simulink model "bh_2dof_NP_LGR_COMPONENT_model"  (R2017a)
settings: Solver=ode45  StartTime=0.0  StopTime=60  FixedStep=0.001  RelTol=1e-7  EnableMultiTasking=on
values from neighbouring files (symbols this model uses):
  theta1_0 = 0    [bh_SIMPARAMS_for_2dof_NP_Control_sim.m]
  theta1_dot_0 = 0    [bh_SIMPARAMS_for_2dof_NP_Control_sim.m]
  theta4_0 = 0    [bh_SIMPARAMS_for_2dof_NP_Control_sim.m]
  theta4_dot_0 = 0    [bh_SIMPARAMS_for_2dof_NP_Control_sim.m]
undefined symbols (not defined in the file or in its folder): b1_damp, b4_damp, g, L1x, L1y, L1z, mass1, mass4, Rturn
settings Model: Creator=bhorton  LastModifiedBy=bhorton
settings SolverCC: ZeroCrossAlgorithm=Adaptive
settings OptimizationCC: LifeSpan=inf
settings DebuggingCC: SFUnexpectedBacktrackingDiag=warning  SFNoUnconditionalDefaultTransitionDiag=warning  SFExecutionAtInitializationDiag=none
settings GRTTargetCC: TargetLangStandard=C89/C90 (ANSI)
settings ConfigComp: CovMetricSettings=dw  CovHtmlReporting=on  CovSaveCumulativeToWorkspaceVar=on  CovSaveSingleToWorkspaceVar=on  CovExternalEMLEnable=off
settings SimscapeCC: SimscapeLogDataHistory=10000  SelectedTab=Simscape Multibody
settings ExplorerConfigSet: InternalSimMechanicsExplorerSettings="<ExplorerConfiguration><canonicalview>default</canonicalview><AnimationSetting><BasePlaybackSpeed>1.0</BasePlaybackSpeed><PlaybackSpeedFactor>1.0</PlaybackSpeedFactor></AnimationSetting><TilePanel><TileInfo><Tiles Columns=\"2\" Count=\"4\" Rows=\"2\"><Column Left=\"2\" Weight=\"0.4997\"/><Column Left=\"761\" Weight=\"0.5003\"/><Column Left=\"1521\"/><Row Top=\"2\" Weight=\"0.4995\"/><Row Top=\"476\" Weight=\"0.5005\"/><Row Top=\"951\"/><Tile Height=\"1\" Width=\"1\" X=\"0\" Y=\"0\"/><Tile Height=\"1\" Width=\"1\" X=\"0\" Y=\"1\"/><Tile Height=\"1\" Width=\"1\" X=\"1\" Y=\"0\"/><Tile Height=\"1\" Width=\"1\" X=\"1\" Y=\"1\"/></Tiles></TileInfo><SceneInfo><SceneViewer><BGColor><R>0.60000002384185791</R><G>0.60000002384185791</G><B>0.60000002384185791</B></BGColor><Camera><DoPerspective>off</DoPerspective><Position><X>0</X><Y>-1.4608099072997489</Y><Z>-0.57289350032806285</Z></Position><Center><X>0</X><Y>0.46399667501581587</Y><Z>-0.57289350032806285</Z></Center><Up><X>0</X><Y>-0</Y><Z>1</Z></Up><ViewLimDist>1</ViewLimDist><YLim>0.6047525054216385</YLim><XLim>0.97540726680909429</XLim></Camera></SceneViewer><SceneViewer><BGColor><R>0.60000002384185791</R><G>0.60000002384185791</G><B>0.60000002384185791</B></BGColor><Camera><DoPerspective>off</DoPerspective><Position><X>0.015927683572912424</X><Y>0.0885583895662721</Y><Z>1.3002562391579151</Z></Position><Center><X>0.015927683572912424</X><Y>0.0885583895662721</Y><Z>-0.5728934407234183</Z></Center><Up><X>0</X><Y>1</Y><Z>-0</Z></Up><ViewLimDist>1</ViewLimDist><YLim>0.53016432464122776</YLim><XLim>0.85326876283459407</XLim></Camera></SceneViewer><SceneViewer><BGColor><R>0.60000002384185791</R><G>0.60000002384185791</G><B>0.60000002384185791</B></BGColor><Camera><DoPerspective>off</DoPerspective><Position><X>1.3697650679051876</X><Y>0.46399664521349349</Y><Z>-0.57289350032806308</Z></Position><Center><X>5.5511151231257827e-17</X><Y>0.46399664521349349</Y><Z>-0.57289350032806308</Z></Center><Up><X>-0</X><Y>0</Y><Z>1</Z></Up><ViewLimDist>1</ViewLimDist><YLim>0.6047525054216385</YLim><XLim>0.9767078098315064</XLim></Camera></SceneViewer><SceneViewer><BGColor><R>0.60000002384185791</R><G>0.60000002384185791</G><B>0.60000002384185791</B></BGColor><Camera><DoPerspective>off</DoPerspective><Position><X>1.0233612252488975</X><Y>-0.57562481311748281</Y><Z>0.47679029183024879</Z></Position><Center><X>-0.00096063421143327554</X><Y>0.44869704634284813</Y><Z>-0.54753156763008215</Z></Center><Up><X>-0.40824829046386307</X><Y>0.40824829046386307</Y><Z>0.81649658092772615</Z></Up><ViewLimDist>1</ViewLimDist><YLim>0.31343533396720885</YLim><XLim>0.50512861761668204</XLim></Camera></SceneViewer></SceneInfo></TilePanel><MechEditorPanel><Cameras/><GfxPanelCameraMap/><VideoCreator><PlaybackSpeedRatio>1.0</PlaybackSpeedRatio><FrameRate>30</FrameRate><VideoFormat>Motion JPEG AVI</VideoFormat><FrameSize>auto</FrameSize></VideoCreator></MechEditorPanel></ExplorerConfiguration>"

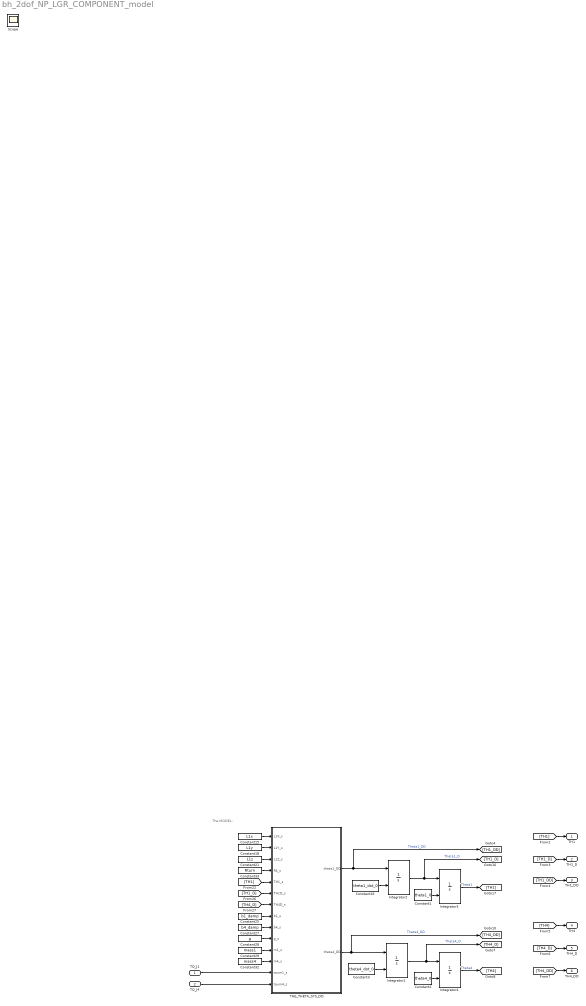
== system bh_2dof_NP_LGR_COMPONENT_model ==
  note: The MODEL:
  "TQ_J1 " : Inport
  TQ_J4 : Inport  Port=2
  Constant1 : Constant  Value=theta1_0
  Constant15 : Constant  Value=L1x
  Constant16 : Constant  Value=theta1_dot_0
  Constant18 : Constant  Value=L1y
  Constant2 : Constant  Value=theta4_0
  Constant21 : Constant  Value=L1z
  Constant25 : Constant  Value=b1_damp
  Constant27 : Constant  Value=b4_damp
  Constant28 : Constant  Value=g
  Constant29 : Constant  Value=mass1
  Constant3 : Constant  Value=theta4_dot_0
  Constant32 : Constant  Value=mass4
  Constant33 : Constant  Value=Rturn
  Integrator{1..4} (4 alike) : Integrator  InitialConditionSource=external
  THE_THETA_SYS_DD : MATLAB Function  TreatAsAtomicUnit=on
  TH1 : Outport
  TH1_D : Outport  Port=2
  TH1_DD : Outport  Port=3
  TH4 : Outport  Port=4
  TH4_D : Outport  Port=5
  TH4_DD : Outport  Port=6
  Scope : Scope
  wires:
  [TH1] -> TH1/1
  [TH1_D] -> TH1_D/1
  [TH1_DD] -> TH1_DD/1
  [TH4_DD] -> TH4_DD/1
  [TH4_D] -> TH4_D/1
  [TH4] -> TH4/1
  Constant32/1 -> THE_THETA_SYS_DD/12(m4_s)
  Constant29/1 -> THE_THETA_SYS_DD/11(m1_s)
  Constant28/1 -> THE_THETA_SYS_DD/10(g_s)
  Constant27/1 -> THE_THETA_SYS_DD/9(b4_s)
  Constant25/1 -> THE_THETA_SYS_DD/8(b1_s)
  [TH4_D] -> THE_THETA_SYS_DD/7(TH4D_s)
  [TH1_D] -> THE_THETA_SYS_DD/6(TH1D_s)
  [TH1] -> THE_THETA_SYS_DD/5(TH1_s)
  Constant33/1 -> THE_THETA_SYS_DD/4(R4_s)
  Constant21/1 -> THE_THETA_SYS_DD/3(L1Z_s)
  Constant18/1 -> THE_THETA_SYS_DD/2(L1Y_s)
  Constant15/1 -> THE_THETA_SYS_DD/1(L1X_s)
  TQ_J4/1 -> THE_THETA_SYS_DD/14(taum4_s)
  "TQ_J1 "/1 -> THE_THETA_SYS_DD/13(taum1_s)
  THE_THETA_SYS_DD/1(theta1_DD) -> [TH1_DD], Integrator2/1  "Theta1_DD"
  Constant1/1 -> Integrator3/2
  Constant16/1 -> Integrator2/2
  Integrator3/1 -> [TH1]  "Theta1"
  Integrator2/1 -> [TH1_D], Integrator3/1  "Theta1_D"
  THE_THETA_SYS_DD/2(theta4_DD) -> Integrator1/1, [TH4_DD]  "Theta4_DD"
  Integrator1/1 -> [TH4_D], Integrator4/1  "Theta4_D"
  Constant2/1 -> Integrator4/2
  Constant3/1 -> Integrator1/2
  Integrator4/1 -> [TH4]  "Theta4"

== matlab function bh_2dof_NP_LGR_COMPONENT_model/THE_THETA_SYS_DD ==
  data: L1X_s input; theta1_DD output; L1Y_s input; L1Z_s input; R4_s input; TH1_s input; TH1D_s input; TH4D_s input; b1_s input; b4_s input; g_s input; m1_s input; m4_s input; taum1_s input; taum4_s input; theta4_DD output
function [theta1_DD,theta4_DD] = THE_THETA_SYS_DD(L1X_s,L1Y_s,L1Z_s,R4_s,TH1_s,TH1D_s,TH4D_s,b1_s,b4_s,g_s,m1_s,m4_s,taum1_s,taum4_s)
%#codegen

%    This function was generated by the Symbolic Math Toolbox version 7.2.
%    19-Jul-2017 16:42:27

theta1_DD = (taum1_s.*1.2e1-TH1D_s.*b1_s.*1.2e1-L1Y_s.*g_s.*m1_s.*cos(TH1_s).*6.0-L1Y_s.^2.*TH4D_s.^2.*m1_s.*sin(TH1_s.*2.0).*2.0+L1Z_s.^2.*TH4D_s.^2.*m1_s.*sin(TH1_s.*2.0).*(1.0./2.0))./(L1Y_s.^2.*m1_s.*4.0+L1Z_s.^2.*m1_s);
if nargout > 1
    theta4_DD = (taum4_s.*2.4e1-TH4D_s.*b4_s.*2.4e1+L1Y_s.^2.*TH1D_s.*TH4D_s.*m1_s.*sin(TH1_s.*2.0).*8.0-L1Z_s.^2.*TH1D_s.*TH4D_s.*m1_s.*sin(TH1_s.*2.0).*2.0)./(L1X_s.^2.*m1_s.*2.0+L1Y_s.^2.*m1_s.*4.0+L1Z_s.^2.*m1_s+R4_s.^2.*m4_s.*1.2e1+L1Y_s.^2.*m1_s.*cos(TH1_s.*2.0).*4.0-L1Z_s.^2.*m1_s.*cos(TH1_s.*2.0));
end
